simulink library "HANcoder_STM32_Target2018b"  (R2018b)
settings: Solver=ode45  StartTime=0.0  StopTime=10.0  RelTol=1e-3  EnableMultiTasking=on
libraries: simulink x3
(part 7 of 7)

== system HANcoder_STM32_Target2018b/STM32-P405/Digital Outputs/Digital Output ==
  In1 : Inport
  Level-2 M-file S-Function : M-S-Function  FunctionName=sfcn_digital_out  Parameters=tsamp, pinID, config
  wires:
  In1/1 -> Level-2 M-file S-Function/1

== system HANcoder_STM32_Target2018b/STM32-P405/Error Handling/Clear errors ==
  Trigger : TriggerPort  VariantControl=(inherit)
  Level-2 M-file S-Function : M-S-Function  FunctionName=sfcn_controller_error_clearerrors  Parameters=eepromString

== system HANcoder_STM32_Target2018b/STM32-P405/Error Handling/Delete error ==
  Trigger : TriggerPort  VariantControl=(inherit)
  Constant : Constant  OutDataTypeStr=uint8  SampleTime=-1
  Gnd1 : Ground
  Gnd2 : Ground
  Level-2 M-file S-Function : M-S-Function  FunctionName=sfcn_controller_error_deleteerror_in  Parameters=useInPorts, errorID, para
  wires:
  Gnd2/1 -> Level-2 M-file S-Function/2
  Gnd1/1 -> Level-2 M-file S-Function/1
  Constant/1 -> Level-2 M-file S-Function/3

== system HANcoder_STM32_Target2018b/STM32-P405/Error Handling/Read active error ==
  In1 : Inport
  Level-2 M-file S-Function : M-S-Function  FunctionName=sfcn_controller_error_readerror  Parameters=tsamp
  numbers : Outport
  code : Outport  Port=2
  parameter : Outport  Port=3
  Xtimes : Outport  Port=4
  timestamp : Outport  Port=5
  wires:
  Level-2 M-file S-Function/1 -> numbers/1
  Level-2 M-file S-Function/2 -> code/1
  Level-2 M-file S-Function/3 -> parameter/1
  Level-2 M-file S-Function/4 -> Xtimes/1
  Level-2 M-file S-Function/5 -> timestamp/1
  In1/1 -> Level-2 M-file S-Function/1

== system HANcoder_STM32_Target2018b/STM32-P405/Error Handling/Read stored error ==
  In1 : Inport
  Level-2 M-file S-Function : M-S-Function  FunctionName=sfcn_controller_error_readerror  Parameters=tsamp
  numbers : Outport
  code : Outport  Port=2
  parameter : Outport  Port=3
  Xtimes : Outport  Port=4
  timestamp : Outport  Port=5
  wires:
  In1/1 -> Level-2 M-file S-Function/1
  Level-2 M-file S-Function/5 -> timestamp/1
  Level-2 M-file S-Function/4 -> Xtimes/1
  Level-2 M-file S-Function/3 -> parameter/1
  Level-2 M-file S-Function/2 -> code/1
  Level-2 M-file S-Function/1 -> numbers/1

== system HANcoder_STM32_Target2018b/STM32-P405/Error Handling/Search active error ==
  In1 : Inport
  In2 : Inport  Port=2
  Level-2 M-file S-Function : M-S-Function  FunctionName=sfcn_controller_error_searcherror  Parameters=tsamp
  occurrence : Outport
  timestamp : Outport  Port=2
  wires:
  In1/1 -> Level-2 M-file S-Function/1
  In2/1 -> Level-2 M-file S-Function/2
  Level-2 M-file S-Function/1 -> occurrence/1
  Level-2 M-file S-Function/2 -> timestamp/1

== system HANcoder_STM32_Target2018b/STM32-P405/Error Handling/Search stored error ==
  In1 : Inport
  In2 : Inport  Port=2
  Level-2 M-file S-Function : M-S-Function  FunctionName=sfcn_controller_error_searcherror  Parameters=tsamp
  occurrence : Outport
  timestamp : Outport  Port=2
  wires:
  Level-2 M-file S-Function/2 -> timestamp/1
  Level-2 M-file S-Function/1 -> occurrence/1
  In2/1 -> Level-2 M-file S-Function/2
  In1/1 -> Level-2 M-file S-Function/1

== system HANcoder_STM32_Target2018b/STM32-P405/Error Handling/Store error  ==
  Trigger : TriggerPort  VariantControl=(inherit)
  Gnd1 : Ground
  Gnd2 : Ground
  Level-2 M-file S-Function : M-S-Function  FunctionName=sfcn_controller_error_storeerror_in  Parameters=useInPorts, errorCode, parameter
  wires:
  Gnd1/1 -> Level-2 M-file S-Function/1
  Gnd2/1 -> Level-2 M-file S-Function/2

== system HANcoder_STM32_Target2018b/STM32-P405/Error Handling/Total Errors ==
  Level-2 M-file S-Function : M-S-Function  FunctionName=sfcn_controller_error_totalerrors  Parameters=eepromString, tsamp
  Out1 : Outport
  Out2 : Outport  Port=2
  wires:
  Level-2 M-file S-Function/1 -> Out1/1
  Level-2 M-file S-Function/2 -> Out2/1

== system HANcoder_STM32_Target2018b/STM32-P405/File Logger/File Logger Close ==
  Trigger : TriggerPort  VariantControl=(inherit)
  Level-2 M-file S-Function : M-S-Function  FunctionName=sfcn_filelogger_close

== system HANcoder_STM32_Target2018b/STM32-P405/File Logger/File Logger Init ==
  (Re)start : TriggerPort  VariantControl=(inherit)
  Level-2 M-file S-Function : M-S-Function  FunctionName=sfcn_filelogger_init

== system HANcoder_STM32_Target2018b/STM32-P405/File Logger/File Logger Signal ==
  In1 : Inport
  Level-2 M-file S-Function : M-S-Function  FunctionName=sfcn_filelogger_signal  Parameters=dataType
  wires:
  In1/1 -> Level-2 M-file S-Function/1

== system HANcoder_STM32_Target2018b/STM32-P405/Memory/EEPROM ==
  Erase EEPROM : Subsystem  Tag=HANcoder_TARGET_STM32_P405  mask(Erase EEPROM){}
      mask help:
      | Function
      | ========
      | Erases all identifier values from EEPROM.
      |
      | Triggerport
      | ===========
      | Connect the port to a trigger source to execute the block only when necessary.
      mask init:
      | sfcn_eeprom_clear_mcb();
      settings: MoveFcn=drawLogos
      mask Display: fprintf('Erase EEPROM');patch([80 86 86],[8 14 2],[1 0 0]);patch([88 88 94],[14 2 8],[0 0 0.35]);
  Read from EEPROM : Subsystem  Tag=HANcoder_TARGET_STM32_P405  mask(Read from EEPROM){tsamp=-1}
      mask prompts: tsamp "Sample time"
      mask help:
      | Function
      | ========
      | Read a value from the specified EEPROM identifier.
      |
      | Inport
      | ==========
      | id:
      |   The EEPROM identifier. This input is of type UINT8 and can have a value
      |   between 0..255 to select one of the 256 supported application specific
      |   identifiers.
      |
      | Outport
      | =======
      | value:
      |   The value read from the EEPROM identifier. This output is of type UINT16.
      mask init:
      | sfcn_eeprom_read_mcb();
      settings: MoveFcn=drawLogos
      mask Display:
      | fprintf('Read from EEPROM');
      | port_label('input', 1, 'id');
      | port_label('output', 1, 'value');patch([150 156 156],[8 14 2],[1 0 0]);patch([158 158 164],[14 2 8],[0 0 0.35]);
  Save EEPROM : Subsystem  Tag=HANcoder_TARGET_STM32_P405  mask(Save EEPROM){}
      mask help:
      | Function
      | ========
      | The STM32 controller does not have dedicated EEPROM on-chip. All EEPROM
      | write, read and erase operations are therefore performed in a RAM buffer.
      | To make sure RAM buffer contents are still valid after a power-off, its
      | contents needs to be save in flash EEPROM, which is achieved with this
      | block. This is typically called during the software shutdown sequence,
      | right before power off.
      |
      | Triggerport
      | ===========
      | Connect the port to a trigger source to execute the block only when necessary.
      mask init:
      | sfcn_eeprom_save_mcb();
      settings: MoveFcn=drawLogos
      mask Display: fprintf('Save EEPROM');patch([80 86 86],[8 14 2],[1 0 0]);patch([88 88 94],[14 2 8],[0 0 0.35]);
  Write to EEPROM : Subsystem  Tag=HANcoder_TARGET_STM32_P405  mask(Write to EEPROM){tsamp=-1}
      mask prompts: tsamp "Sample time"
      mask help:
      | Function
      | ========
      | Write the value to the specified EEPROM identifier.
      |
      | Inport
      | ==========
      | id:
      |   The EEPROM identifier. This input is of type UINT8 and can have a value
      |   between 0..255 to select one of the 256 supported application specific
      |   identifiers.
      | value:
      |   The value to write to the EEPROM identifier. This input is of type UINT16.
      mask init:
      | sfcn_eeprom_write_mcb();
      settings: MoveFcn=drawLogos
      mask Display:
      | fprintf('Write to EEPROM');
      | port_label('input', 1, 'id');
      | port_label('input', 2, 'value');patch([150 156 156],[8 14 2],[1 0 0]);patch([158 158 164],[14 2 8],[0 0 0.35]);

== system HANcoder_STM32_Target2018b/STM32-P405/PWM Outputs/PWM Duty Cycle ==
  In1 : Inport
  Level-2 M-file S-Function : M-S-Function  FunctionName=sfcn_pwmout_setduty  Parameters=tsamp
  wires:
  In1/1 -> Level-2 M-file S-Function/1

== system HANcoder_STM32_Target2018b/STM32-P405/PWM Outputs/PWM Init ==
  S-Function : S-Function  FunctionName=sfcn_pwmout_init  SFunctionDeploymentMode=off  EnableBusSupport=off
  Term1 : Terminator
  wires:
  S-Function/1 -> Term1/1

== system HANcoder_STM32_Target2018b/STM32-P405/SPI/SPI master init ==
  Level-2 M-file S-Function : M-S-Function  FunctionName=sfcn_spi_master_init

== system HANcoder_STM32_Target2018b/STM32-P405/SPI/SPI master transfer ==
  In1 : Inport
  Level-2 M-file S-Function : M-S-Function  FunctionName=sfcn_spi_master_transfer  Parameters=tsamp
  Out1 : Outport
  wires:
  In1/1 -> Level-2 M-file S-Function/1
  Level-2 M-file S-Function/1 -> Out1/1

== system HANcoder_STM32_Target2018b/STM32-P405/System Config/Base Sample Time config ==
  note: This constant and terminator block introduces the base sample time,
      | set in Base Sample Time config block, to the model. Blocks  with inherited [-1]
      | sample time wich are not connected to blocks with specifically set sample times
      | will use this value. This block also sets the fixed step time parameter in the Simulink Solver.
      | This works during initialization of simulation or build.
  Level-2 M-file S-Function : M-S-Function  FunctionName=sfcn_base_sample_time  Parameters=baseSampleTime, extraStack
  SampleTimeCrowBar : Constant  InitFcn=|  VectorParams1D=off  OutDataTypeStr=boolean  SampleTime=0.01
      | SampleTimeMiliSeconds = get_param(find_system(bdroot, 'LookUnderMasks', 'all', 'FollowLinks', 'off',  'Name', 'Base Sample Time config'), 'baseSampleTime');
      |                                                                                                                                                             
      | SampleTimeSeconds = str2num(SampleTimeMiliSeconds{1,1})/1000;                                                                                               
      |                                                                                                                                                             
      | set_param(bdroot, 'FixedStep', num2str(SampleTimeSeconds));                                                                                                 
      |                                                                                                                                                             
      | set_param(gcb, 'SampleTime', num2str(get_param(bdroot, 'FixedStep')));                                                                                      
      | clear SampleTimeSeconds SampleTimeMiliSeconds
  Terminator : Terminator
  wires:
  SampleTimeCrowBar/1 -> Terminator/1

== system HANcoder_STM32_Target2018b/STM32-P405/System Config/Build settings ==

== system HANcoder_STM32_Target2018b/STM32-P405/System Config/CAN config ==
  Level-2 M-file S-Function : M-S-Function  FunctionName=sfcn_can_config

== system HANcoder_STM32_Target2018b/STM32-P405/System Config/Custom ID config ==
  Level-2 M-file S-Function : M-S-Function  RequirementInfo={}  FunctionName=sfcn_custom_version_config  Parameters=softID

== system HANcoder_STM32_Target2018b/STM32-P405/System Config/XCP on CAN config ==
  Level-2 M-file S-Function : M-S-Function  RequirementInfo={} %GIDa_75ebdf1d_e085_4bd4_9cf7_36846954f0a6  FunctionName=sfcn_can_xcp_config  Parameters=canBus, croID, dtoID

== system HANcoder_STM32_Target2018b/STM32-P405/System Config/XCP on USB config ==
  Level-2 M-file S-Function : M-S-Function  RequirementInfo={} %GIDa_75ebdf1d_e085_4bd4_9cf7_36846954f0a6  FunctionName=sfcn_usb_xcp_config

== system HANcoder_STM32_Target2018b/STM32-P405/System Management/Enter Critical Section ==
  Level-2 M-file S-Function : M-S-Function  FunctionName=sfcn_critical_enter  Parameters=tsamp

== system HANcoder_STM32_Target2018b/STM32-P405/System Management/Exit Critical Section ==
  Level-2 M-file S-Function : M-S-Function  FunctionName=sfcn_critical_exit  Parameters=tsamp

== system HANcoder_STM32_Target2018b/STM32-P405/System Management/Get CPU load ==
  Level-2 M-file S-Function : M-S-Function  FunctionName=sfcn_controller_cpu_getload  Parameters=tsamp, mode
  Out1 : Outport
  wires:
  Level-2 M-file S-Function/1 -> Out1/1

== system HANcoder_STM32_Target2018b/STM32-P405/System Management/Get free Heap ==
  Level-2 M-file S-Function : M-S-Function  FunctionName=sfcn_controller_getheap  Parameters=tsamp
  Out1 : Outport
  wires:
  Level-2 M-file S-Function/1 -> Out1/1

== system HANcoder_STM32_Target2018b/STM32-P405/System Management/Get free Stack ==
  Level-2 M-file S-Function : M-S-Function  FunctionName=sfcn_controller_getstack  Parameters=tsamp, taskIdx
  Out1 : Outport
  wires:
  Level-2 M-file S-Function/1 -> Out1/1

== system HANcoder_STM32_Target2018b/STM32-P405/System Management/Reset ECU ==
  Trigger : TriggerPort  VariantControl=(inherit)
  Level-2 M-file S-Function : M-S-Function  FunctionName=sfcn_controller_reset

== system HANcoder_STM32_Target2018b/STM32-P405/Timer Inputs/Quadrature Encoder Get ==
  Data Type Conversion : DataTypeConversion  OutDataTypeStr=boolean
  Detect Increase : simulink/Logic and Bit Operations/Detect Increase  vinit=0.0  OutDataTypeStr=uint8
  Gnd1 : Ground
  Level-2 M-file S-Function : M-S-Function  FunctionName=sfcn_quad_encoder_get  Parameters=tsamp, moduleID
  Out1 : Outport
  wires:
  Data Type Conversion/1 -> Level-2 M-file S-Function/1
  Detect Increase/1 -> Data Type Conversion/1
  Gnd1/1 -> Detect Increase/1
  Level-2 M-file S-Function/1 -> Out1/1

== system HANcoder_STM32_Target2018b/STM32-P405/Timer Inputs/Timer Input Get ==
  Level-2 M-file S-Function : M-S-Function  FunctionName=sfcn_timein_get  Parameters=tsamp
  Out1 : Outport
  Out2 : Outport  Port=2
  Out3 : Outport  Port=3
  Out4 : Outport  Port=4
  Out5 : Outport  Port=5
  Out6 : Outport  Port=6
  Out7 : Outport  Port=7
  wires:
  Level-2 M-file S-Function/1 -> Out1/1
  Level-2 M-file S-Function/2 -> Out2/1
  Level-2 M-file S-Function/3 -> Out3/1
  Level-2 M-file S-Function/4 -> Out4/1
  Level-2 M-file S-Function/5 -> Out5/1
  Level-2 M-file S-Function/6 -> Out6/1
  Level-2 M-file S-Function/7 -> Out7/1

== system HANcoder_STM32_Target2018b/STM32-P405/Timer Inputs/Timer Input IRQ ==
  S-Function : S-Function  FunctionName=sfcn_timein_irq  SFunctionDeploymentMode=off  EnableBusSupport=off
  Out1 : Outport
  wires:
  S-Function/1 -> Out1/1

== system HANcoder_STM32_Target2018b/STM32-P405/Timer Outputs/Compare Event IRQ ==
  S-Function : S-Function  FunctionName=sfcn_timeout_event_irq  SFunctionDeploymentMode=off  EnableBusSupport=off
  Out1 : Outport
  wires:
  S-Function/1 -> Out1/1

== system HANcoder_STM32_Target2018b/STM32-P405/Timer Outputs/Get Free Running Counter ==
  Level-2 M-file S-Function : M-S-Function  FunctionName=sfcn_timeout_getrunningcounter  Parameters=tsamp
  Out1 : Outport
  wires:
  Level-2 M-file S-Function/1 -> Out1/1

== system HANcoder_STM32_Target2018b/STM32-P405/Timer Outputs/Get Last Event Counter ==
  Level-2 M-file S-Function : M-S-Function  FunctionName=sfcn_timeout_getlasteventcounter  Parameters=tsamp
  Out1 : Outport
  wires:
  Level-2 M-file S-Function/1 -> Out1/1

== system HANcoder_STM32_Target2018b/STM32-P405/Timer Outputs/Output Compare Init ==
  S-Function : S-Function  FunctionName=sfcn_timeout_init  SFunctionDeploymentMode=off  EnableBusSupport=off
  Term1 : Terminator
  wires:
  S-Function/1 -> Term1/1

== system HANcoder_STM32_Target2018b/STM32-P405/Timer Outputs/Reset Free Running Counter ==
  Trigger : TriggerPort  VariantControl=(inherit)
  Level-2 M-file S-Function : M-S-Function  FunctionName=sfcn_timeout_resetcounter

== system HANcoder_STM32_Target2018b/STM32-P405/Timer Outputs/Schedule Compare Event ==
  In1 : Inport
  In2 : Inport  Port=2
  Level-2 M-file S-Function : M-S-Function  FunctionName=sfcn_timeout_scheduleevent  Parameters=tsamp
  wires:
  In2/1 -> Level-2 M-file S-Function/2
  In1/1 -> Level-2 M-file S-Function/1

== system HANcoder_STM32_Target2018b/STM32-P405/UART/UART init ==
  Level-2 M-file S-Function : M-S-Function  FunctionName=sfcn_uart_init
  Term1 : Terminator
  wires:
  Level-2 M-file S-Function/1 -> Term1/1

== system HANcoder_STM32_Target2018b/STM32-P405/UART/UART receive ==
  Level-2 M-file S-Function : M-S-Function  FunctionName=sfcn_uart_receive  Parameters=tsamp
  Term1 : Terminator
  Out1 : Outport
  wires:
  Level-2 M-file S-Function/2 -> Term1/1
  Level-2 M-file S-Function/1 -> Out1/1

== system HANcoder_STM32_Target2018b/STM32-P405/UART/UART receive buffer status ==
  Level-2 M-file S-Function : M-S-Function  FunctionName=sfcn_uart_receive_size  Parameters=tsamp
  Out1 : Outport
  wires:
  Level-2 M-file S-Function/1 -> Out1/1

== system HANcoder_STM32_Target2018b/STM32-P405/UART/UART send ==
  In1 : Inport
  Level-2 M-file S-Function : M-S-Function  FunctionName=sfcn_uart_send  Parameters=tsamp
  Term1 : Terminator
  wires:
  In1/1 -> Level-2 M-file S-Function/1
  Level-2 M-file S-Function/1 -> Term1/1

== system HANcoder_STM32_Target2018b/STM32-P405/UDS/UDS Get Key ==
  S-Function : M-S-Function  FunctionName=sfcn_uds_get_key  Parameters=tsamp
  Out1 : Outport
  wires:
  S-Function/1 -> Out1/1

== system HANcoder_STM32_Target2018b/STM32-P405/UDS/UDS Get Seed ==
  S-Function : M-S-Function  FunctionName=sfcn_uds_get_seed  Parameters=tsamp
  Out1 : Outport
  wires:
  S-Function/1 -> Out1/1

== system HANcoder_STM32_Target2018b/STM32-P405/UDS/UDS Get Seed Event ==
  S-Function : S-Function  FunctionName=sfcn_uds_get_seed_event  SFunctionDeploymentMode=off  EnableBusSupport=off
  Out1 : Outport
  wires:
  S-Function/1 -> Out1/1

== system HANcoder_STM32_Target2018b/STM32-P405/UDS/UDS Init ==
  S-Function : M-S-Function  FunctionName=sfcn_uds_init

== system HANcoder_STM32_Target2018b/STM32-P405/UDS/UDS Set Key Verfied ==
  In1 : Inport
  S-Function : M-S-Function  FunctionName=sfcn_uds_set_key_verified  Parameters=tsamp
  wires:
  In1/1 -> S-Function/1

== system HANcoder_STM32_Target2018b/STM32-P405/UDS/UDS Set Seed ==
  In1 : Inport
  S-Function : M-S-Function  FunctionName=sfcn_uds_set_seed  Parameters=tsamp
  wires:
  In1/1 -> S-Function/1

== system HANcoder_STM32_Target2018b/STM32-P405/UDS/UDS Verify Key Event ==
  S-Function : S-Function  FunctionName=sfcn_uds_verify_key_event  SFunctionDeploymentMode=off  EnableBusSupport=off
  Out1 : Outport
  wires:
  S-Function/1 -> Out1/1

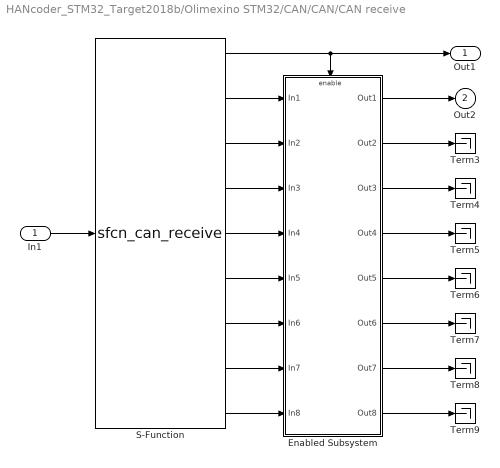
== system HANcoder_STM32_Target2018b/Olimexino STM32/CAN/CAN/CAN receive ==
  In1 : Inport
  Enabled Subsystem : Subsystem  TreatAsAtomicUnit=on
  S-Function : M-S-Function  FunctionName=sfcn_can_receive  Parameters=tsamp, canBus, outputNumber, dataType, byteOrder
  Term{3..9} (7 alike) : Terminator
  Out1 : Outport
  Out2 : Outport  Port=2
  wires:
  In1/1 -> S-Function/1
  S-Function/1 -> Enabled Subsystem/Enable, Out1/1
  S-Function/6 -> Enabled Subsystem/5(In5)
  S-Function/5 -> Enabled Subsystem/4(In4)
  S-Function/9 -> Enabled Subsystem/8(In8)
  S-Function/2 -> Enabled Subsystem/1(In1)
  S-Function/3 -> Enabled Subsystem/2(In2)
  S-Function/4 -> Enabled Subsystem/3(In3)
  S-Function/8 -> Enabled Subsystem/7(In7)
  S-Function/7 -> Enabled Subsystem/6(In6)
  Enabled Subsystem/1(Out1) -> Out2/1
  Enabled Subsystem/2(Out2) -> Term3/1
  Enabled Subsystem/3(Out3) -> Term4/1
  Enabled Subsystem/4(Out4) -> Term5/1
  Enabled Subsystem/5(Out5) -> Term6/1
  Enabled Subsystem/6(Out6) -> Term7/1
  Enabled Subsystem/7(Out7) -> Term8/1
  Enabled Subsystem/8(Out8) -> Term9/1

== system HANcoder_STM32_Target2018b/Olimexino STM32/CAN/CAN/CAN receive packed ==
  Enabled Subsystem : Subsystem  TreatAsAtomicUnit=on
  S-Function : M-S-Function  FunctionName=sfcn_can_receive_packed  Parameters=tsamp, canBus, canID
  Out1 : Outport
  Out2 : Outport  Port=2
  wires:
  S-Function/1 -> Enabled Subsystem/Enable, Out1/1
  S-Function/2 -> Enabled Subsystem/1(In1)
  Enabled Subsystem/1(Out1) -> Out2/1

== system HANcoder_STM32_Target2018b/Olimexino STM32/CAN/CAN/CAN send ==
  In1 : Inport
  In2 : Inport  Port=2
  In3 : Inport  Port=3
  In4 : Inport  Port=4
  In5 : Inport  Port=5
  In6 : Inport  Port=6
  In7 : Inport  Port=7
  In8 : Inport  Port=8
  In9 : Inport  Port=9
  S-Function : M-S-Function  FunctionName=sfcn_can_send  Parameters=tsamp, canBus, frameType, inputNumber, dataType, byteOrder
  wires:
  In1/1 -> S-Function/1
  In2/1 -> S-Function/2
  In3/1 -> S-Function/3
  In4/1 -> S-Function/4
  In5/1 -> S-Function/5
  In6/1 -> S-Function/6
  In7/1 -> S-Function/7
  In8/1 -> S-Function/8
  In9/1 -> S-Function/9

== system HANcoder_STM32_Target2018b/Olimexino STM32/CAN/CAN/CAN send packed ==
  In1 : Inport
  S-Function : M-S-Function  FunctionName=sfcn_can_send_packed  Parameters=tsamp, canBus
  wires:
  In1/1 -> S-Function/1

== system HANcoder_STM32_Target2018b/Olimexino STM32/CAN/CANopenNode/CANopenNode Init ==
  S-Function : M-S-Function  FunctionName=sfcn_can_canopennode_init  Parameters=channel

== system HANcoder_STM32_Target2018b/Olimexino STM32/CAN/CANopenNode/CANopenNode OD Read ==
  S-Function : M-S-Function  FunctionName=sfcn_can_canopennode_od_read  Parameters=tsamp, dataType
  Out1 : Outport
  wires:
  S-Function/1 -> Out1/1

== system HANcoder_STM32_Target2018b/Olimexino STM32/CAN/CANopenNode/CANopenNode OD Write ==
  In1 : Inport
  S-Function : M-S-Function  FunctionName=sfcn_can_canopennode_od_write  Parameters=tsamp, dataType
  wires:
  In1/1 -> S-Function/1

== system HANcoder_STM32_Target2018b/Olimexino STM32/Memory/EEPROM/Erase EEPROM ==
  Trigger : TriggerPort  VariantControl=(inherit)
  Level-2 M-file S-Function : M-S-Function  FunctionName=sfcn_eeprom_clear

== system HANcoder_STM32_Target2018b/Olimexino STM32/Memory/EEPROM/Read from EEPROM ==
  In1 : Inport
  Level-2 M-file S-Function : M-S-Function  FunctionName=sfcn_eeprom_read  Parameters=tsamp
  Out1 : Outport
  wires:
  In1/1 -> Level-2 M-file S-Function/1
  Level-2 M-file S-Function/1 -> Out1/1

== system HANcoder_STM32_Target2018b/Olimexino STM32/Memory/EEPROM/Save EEPROM ==
  Trigger : TriggerPort  VariantControl=(inherit)
  Level-2 M-file S-Function : M-S-Function  FunctionName=sfcn_eeprom_save

== system HANcoder_STM32_Target2018b/Olimexino STM32/Memory/EEPROM/Write to EEPROM ==
  In1 : Inport
  In2 : Inport  Port=2
  Level-2 M-file S-Function : M-S-Function  FunctionName=sfcn_eeprom_write  Parameters=tsamp
  wires:
  In1/1 -> Level-2 M-file S-Function/1
  In2/1 -> Level-2 M-file S-Function/2

== system HANcoder_STM32_Target2018b/STM32-E407/CAN/CAN/CAN receive ==
  In1 : Inport
  Enabled Subsystem : Subsystem  TreatAsAtomicUnit=on
  S-Function : M-S-Function  FunctionName=sfcn_can_receive  Parameters=tsamp, canBus, outputNumber, dataType, byteOrder
  Term{3..9} (7 alike) : Terminator
  Out1 : Outport
  Out2 : Outport  Port=2
  wires:
  In1/1 -> S-Function/1
  S-Function/1 -> Enabled Subsystem/Enable, Out1/1
  S-Function/2 -> Enabled Subsystem/1(In1)
  S-Function/3 -> Enabled Subsystem/2(In2)
  Enabled Subsystem/1(Out1) -> Out2/1
  Enabled Subsystem/2(Out2) -> Term3/1
  Enabled Subsystem/3(Out3) -> Term4/1
  Enabled Subsystem/4(Out4) -> Term5/1
  Enabled Subsystem/5(Out5) -> Term6/1
  Enabled Subsystem/6(Out6) -> Term7/1
  Enabled Subsystem/7(Out7) -> Term8/1
  Enabled Subsystem/8(Out8) -> Term9/1
  S-Function/6 -> Enabled Subsystem/5(In5)
  S-Function/7 -> Enabled Subsystem/6(In6)
  S-Function/8 -> Enabled Subsystem/7(In7)
  S-Function/5 -> Enabled Subsystem/4(In4)
  S-Function/4 -> Enabled Subsystem/3(In3)
  S-Function/9 -> Enabled Subsystem/8(In8)

== system HANcoder_STM32_Target2018b/STM32-E407/CAN/CAN/CAN receive packed ==
  Enabled Subsystem : Subsystem  TreatAsAtomicUnit=on
  S-Function : M-S-Function  FunctionName=sfcn_can_receive_packed  Parameters=tsamp, canBus, canID
  Out1 : Outport
  Out2 : Outport  Port=2
  wires:
  S-Function/1 -> Enabled Subsystem/Enable, Out1/1
  S-Function/2 -> Enabled Subsystem/1(In1)
  Enabled Subsystem/1(Out1) -> Out2/1

== system HANcoder_STM32_Target2018b/STM32-E407/CAN/CAN/CAN send ==
  In1 : Inport
  In2 : Inport  Port=2
  In3 : Inport  Port=3
  In4 : Inport  Port=4
  In5 : Inport  Port=5
  In6 : Inport  Port=6
  In7 : Inport  Port=7
  In8 : Inport  Port=8
  In9 : Inport  Port=9
  S-Function : M-S-Function  FunctionName=sfcn_can_send  Parameters=tsamp, canBus, frameType, inputNumber, dataType, byteOrder
  wires:
  In9/1 -> S-Function/9
  In8/1 -> S-Function/8
  In7/1 -> S-Function/7
  In6/1 -> S-Function/6
  In5/1 -> S-Function/5
  In4/1 -> S-Function/4
  In3/1 -> S-Function/3
  In2/1 -> S-Function/2
  In1/1 -> S-Function/1

== system HANcoder_STM32_Target2018b/STM32-E407/CAN/CAN/CAN send packed ==
  In1 : Inport
  S-Function : M-S-Function  FunctionName=sfcn_can_send_packed  Parameters=tsamp, canBus
  wires:
  In1/1 -> S-Function/1

== system HANcoder_STM32_Target2018b/STM32-E407/CAN/CANopenNode/CANopenNode Init ==
  S-Function : M-S-Function  FunctionName=sfcn_can_canopennode_init  Parameters=channel

== system HANcoder_STM32_Target2018b/STM32-E407/CAN/CANopenNode/CANopenNode OD Read ==
  S-Function : M-S-Function  FunctionName=sfcn_can_canopennode_od_read  Parameters=tsamp, dataType
  Out1 : Outport
  wires:
  S-Function/1 -> Out1/1

== system HANcoder_STM32_Target2018b/STM32-E407/CAN/CANopenNode/CANopenNode OD Write ==
  In1 : Inport
  S-Function : M-S-Function  FunctionName=sfcn_can_canopennode_od_write  Parameters=tsamp, dataType
  wires:
  In1/1 -> S-Function/1

== system HANcoder_STM32_Target2018b/STM32-E407/Memory/EEPROM/Erase EEPROM ==
  Trigger : TriggerPort  VariantControl=(inherit)
  Level-2 M-file S-Function : M-S-Function  FunctionName=sfcn_eeprom_clear

== system HANcoder_STM32_Target2018b/STM32-E407/Memory/EEPROM/Read from EEPROM ==
  In1 : Inport
  Level-2 M-file S-Function : M-S-Function  FunctionName=sfcn_eeprom_read  Parameters=tsamp
  Out1 : Outport
  wires:
  Level-2 M-file S-Function/1 -> Out1/1
  In1/1 -> Level-2 M-file S-Function/1

== system HANcoder_STM32_Target2018b/STM32-E407/Memory/EEPROM/Save EEPROM ==
  Trigger : TriggerPort  VariantControl=(inherit)
  Level-2 M-file S-Function : M-S-Function  FunctionName=sfcn_eeprom_save

== system HANcoder_STM32_Target2018b/STM32-E407/Memory/EEPROM/Write to EEPROM ==
  In1 : Inport
  In2 : Inport  Port=2
  Level-2 M-file S-Function : M-S-Function  FunctionName=sfcn_eeprom_write  Parameters=tsamp
  wires:
  In2/1 -> Level-2 M-file S-Function/2
  In1/1 -> Level-2 M-file S-Function/1

== system HANcoder_STM32_Target2018b/STM32-P405/CAN/CAN/CAN receive ==
  In1 : Inport
  Enabled Subsystem : Subsystem  TreatAsAtomicUnit=on
  S-Function : M-S-Function  FunctionName=sfcn_can_receive  Parameters=tsamp, canBus, outputNumber, dataType, byteOrder
  Term{3..9} (7 alike) : Terminator
  Out1 : Outport
  Out2 : Outport  Port=2
  wires:
  In1/1 -> S-Function/1
  S-Function/1 -> Out1/1, Enabled Subsystem/Enable
  S-Function/2 -> Enabled Subsystem/1(In1)
  S-Function/3 -> Enabled Subsystem/2(In2)
  Enabled Subsystem/1(Out1) -> Out2/1
  Enabled Subsystem/2(Out2) -> Term3/1
  Enabled Subsystem/3(Out3) -> Term4/1
  Enabled Subsystem/4(Out4) -> Term5/1
  Enabled Subsystem/5(Out5) -> Term6/1
  Enabled Subsystem/6(Out6) -> Term7/1
  Enabled Subsystem/7(Out7) -> Term8/1
  Enabled Subsystem/8(Out8) -> Term9/1
  S-Function/6 -> Enabled Subsystem/5(In5)
  S-Function/7 -> Enabled Subsystem/6(In6)
  S-Function/8 -> Enabled Subsystem/7(In7)
  S-Function/5 -> Enabled Subsystem/4(In4)
  S-Function/4 -> Enabled Subsystem/3(In3)
  S-Function/9 -> Enabled Subsystem/8(In8)

== system HANcoder_STM32_Target2018b/STM32-P405/CAN/CAN/CAN receive packed ==
  Enabled Subsystem : Subsystem  TreatAsAtomicUnit=on
  S-Function : M-S-Function  FunctionName=sfcn_can_receive_packed  Parameters=tsamp, canBus, canID
  Out1 : Outport
  Out2 : Outport  Port=2
  wires:
  S-Function/1 -> Enabled Subsystem/Enable, Out1/1
  S-Function/2 -> Enabled Subsystem/1(In1)
  Enabled Subsystem/1(Out1) -> Out2/1

== system HANcoder_STM32_Target2018b/STM32-P405/CAN/CAN/CAN send ==
  In1 : Inport
  In2 : Inport  Port=2
  In3 : Inport  Port=3
  In4 : Inport  Port=4
  In5 : Inport  Port=5
  In6 : Inport  Port=6
  In7 : Inport  Port=7
  In8 : Inport  Port=8
  In9 : Inport  Port=9
  S-Function : M-S-Function  FunctionName=sfcn_can_send  Parameters=tsamp, canBus, frameType, inputNumber, dataType, byteOrder
  wires:
  In1/1 -> S-Function/1
  In2/1 -> S-Function/2
  In3/1 -> S-Function/3
  In4/1 -> S-Function/4
  In5/1 -> S-Function/5
  In6/1 -> S-Function/6
  In7/1 -> S-Function/7
  In8/1 -> S-Function/8
  In9/1 -> S-Function/9

== system HANcoder_STM32_Target2018b/STM32-P405/CAN/CAN/CAN send packed ==
  In1 : Inport
  S-Function : M-S-Function  FunctionName=sfcn_can_send_packed  Parameters=tsamp, canBus
  wires:
  In1/1 -> S-Function/1

== system HANcoder_STM32_Target2018b/STM32-P405/CAN/CANopenNode/CANopenNode Init ==
  S-Function : M-S-Function  FunctionName=sfcn_can_canopennode_init  Parameters=channel

== system HANcoder_STM32_Target2018b/STM32-P405/CAN/CANopenNode/CANopenNode OD Read ==
  S-Function : M-S-Function  FunctionName=sfcn_can_canopennode_od_read  Parameters=tsamp, dataType
  Out1 : Outport
  wires:
  S-Function/1 -> Out1/1

== system HANcoder_STM32_Target2018b/STM32-P405/CAN/CANopenNode/CANopenNode OD Write ==
  In1 : Inport
  S-Function : M-S-Function  FunctionName=sfcn_can_canopennode_od_write  Parameters=tsamp, dataType
  wires:
  In1/1 -> S-Function/1

== system HANcoder_STM32_Target2018b/STM32-P405/Memory/EEPROM/Erase EEPROM ==
  Trigger : TriggerPort  VariantControl=(inherit)
  Level-2 M-file S-Function : M-S-Function  FunctionName=sfcn_eeprom_clear

== system HANcoder_STM32_Target2018b/STM32-P405/Memory/EEPROM/Read from EEPROM ==
  In1 : Inport
  Level-2 M-file S-Function : M-S-Function  FunctionName=sfcn_eeprom_read  Parameters=tsamp
  Out1 : Outport
  wires:
  In1/1 -> Level-2 M-file S-Function/1
  Level-2 M-file S-Function/1 -> Out1/1

== system HANcoder_STM32_Target2018b/STM32-P405/Memory/EEPROM/Save EEPROM ==
  Trigger : TriggerPort  VariantControl=(inherit)
  Level-2 M-file S-Function : M-S-Function  FunctionName=sfcn_eeprom_save

== system HANcoder_STM32_Target2018b/STM32-P405/Memory/EEPROM/Write to EEPROM ==
  In1 : Inport
  In2 : Inport  Port=2
  Level-2 M-file S-Function : M-S-Function  FunctionName=sfcn_eeprom_write  Parameters=tsamp
  wires:
  In1/1 -> Level-2 M-file S-Function/1
  In2/1 -> Level-2 M-file S-Function/2

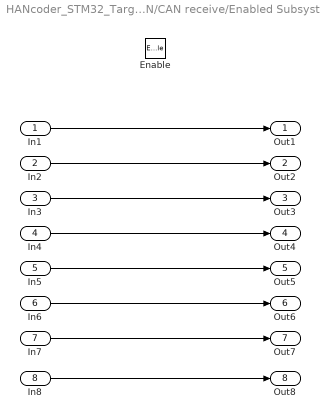
== system HANcoder_STM32_Target2018b/Olimexino STM32/CAN/CAN/CAN receive/Enabled Subsystem ==
  In1 : Inport
  In2 : Inport  Port=2
  In3 : Inport  Port=3
  In4 : Inport  Port=4
  In5 : Inport  Port=5
  In6 : Inport  Port=6
  In7 : Inport  Port=7
  In8 : Inport  Port=8
  Enable : EnablePort
  Out1 : Outport
  Out2 : Outport  Port=2
  Out3 : Outport  Port=3
  Out4 : Outport  Port=4
  Out5 : Outport  Port=5
  Out6 : Outport  Port=6
  Out7 : Outport  Port=7
  Out8 : Outport  Port=8
  wires:
  In1/1 -> Out1/1
  In2/1 -> Out2/1
  In3/1 -> Out3/1
  In4/1 -> Out4/1
  In5/1 -> Out5/1
  In6/1 -> Out6/1
  In7/1 -> Out7/1
  In8/1 -> Out8/1

== system HANcoder_STM32_Target2018b/Olimexino STM32/CAN/CAN/CAN receive packed/Enabled Subsystem ==
  In1 : Inport
  Enable : EnablePort
  Out1 : Outport
  wires:
  In1/1 -> Out1/1

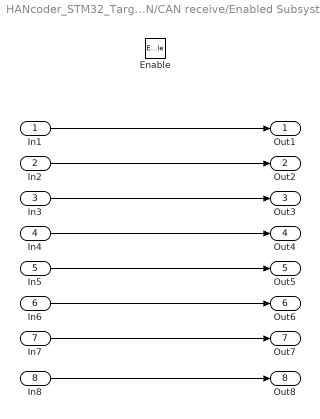
== system HANcoder_STM32_Target2018b/STM32-E407/CAN/CAN/CAN receive/Enabled Subsystem ==
  In1 : Inport
  In2 : Inport  Port=2
  In3 : Inport  Port=3
  In4 : Inport  Port=4
  In5 : Inport  Port=5
  In6 : Inport  Port=6
  In7 : Inport  Port=7
  In8 : Inport  Port=8
  Enable : EnablePort
  Out1 : Outport
  Out2 : Outport  Port=2
  Out3 : Outport  Port=3
  Out4 : Outport  Port=4
  Out5 : Outport  Port=5
  Out6 : Outport  Port=6
  Out7 : Outport  Port=7
  Out8 : Outport  Port=8
  wires:
  In1/1 -> Out1/1
  In2/1 -> Out2/1
  In3/1 -> Out3/1
  In4/1 -> Out4/1
  In5/1 -> Out5/1
  In6/1 -> Out6/1
  In7/1 -> Out7/1
  In8/1 -> Out8/1

== system HANcoder_STM32_Target2018b/STM32-E407/CAN/CAN/CAN receive packed/Enabled Subsystem ==
  In1 : Inport
  Enable : EnablePort
  Out1 : Outport
  wires:
  In1/1 -> Out1/1

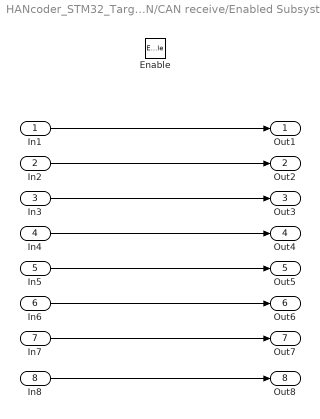
== system HANcoder_STM32_Target2018b/STM32-P405/CAN/CAN/CAN receive/Enabled Subsystem ==
  In1 : Inport
  In2 : Inport  Port=2
  In3 : Inport  Port=3
  In4 : Inport  Port=4
  In5 : Inport  Port=5
  In6 : Inport  Port=6
  In7 : Inport  Port=7
  In8 : Inport  Port=8
  Enable : EnablePort
  Out1 : Outport
  Out2 : Outport  Port=2
  Out3 : Outport  Port=3
  Out4 : Outport  Port=4
  Out5 : Outport  Port=5
  Out6 : Outport  Port=6
  Out7 : Outport  Port=7
  Out8 : Outport  Port=8
  wires:
  In1/1 -> Out1/1
  In2/1 -> Out2/1
  In3/1 -> Out3/1
  In4/1 -> Out4/1
  In5/1 -> Out5/1
  In6/1 -> Out6/1
  In7/1 -> Out7/1
  In8/1 -> Out8/1

== system HANcoder_STM32_Target2018b/STM32-P405/CAN/CAN/CAN receive packed/Enabled Subsystem ==
  In1 : Inport
  Enable : EnablePort
  Out1 : Outport
  wires:
  In1/1 -> Out1/1
